simulink model "python_test"  (R2019b)
settings: Solver=VariableStepAuto  StartTime=0.0  StopTime=10.0  RelTol=1e-3
settings Model: Creator=t2vosx  LastModifiedBy=t2vosx
settings DataIOCC: ReturnWorkspaceOutputs=off
settings DebuggingCC: ArithmeticOperatorsInVariantConditions=warning
settings SFSimCC: CustomCodeUndefinedFunction=UseInterfaceOnly

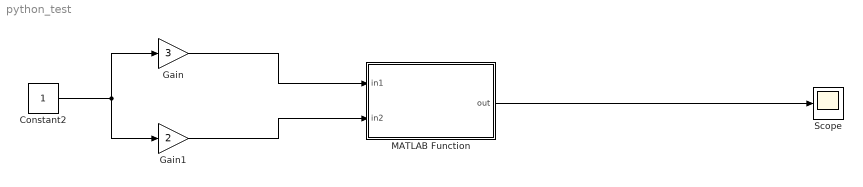
== system python_test ==
  Constant2 : Constant
  Gain : Gain  Gain=3
  Gain1 : Gain  Gain=2
  MATLAB Function : MATLAB Function  TreatAsAtomicUnit=on
  Scope : Scope
  wires:
  Gain/1 -> MATLAB Function/1(in1)
  Gain1/1 -> MATLAB Function/2(in2)
  MATLAB Function/1(out) -> Scope/1
  Constant2/1 -> Gain/1, Gain1/1

== matlab function python_test/MATLAB Function ==
  data: in1 input; out output; in2 input
function out = RunPython(in1, in2)
    out = 0; % Has to be preassigned, otherwise Simulink throws an error
    coder.extrinsic('py.Example.test') % Python functions have to be run extrinsically, meaning no C code generated
    out = py.Example.test(in1,in2);
end
